simulink model "ISP"  (R2022b)
settings: configuration reference "ERT" (kept outside this file)
undefined symbols (not defined in the file): DFC, ECM, facAdc2ubr_C, facNCtrlRateLim_C, FID, IsRate_C, ki_C, tauIsHeatPnt_C, tauOscDrvTrn_C, tInvMax_C, tInvMin_C, trqDmpSta_C, Ts_10ms, Ts_1ms, tStrMax_C, tStrMin_C, ubrMax_C, ubrMin_C, vdd5Max_C, vdd5Min_C
libraries: simulink x18, DSMLib x17, MathLib x10
settings Model: Creator=M00039784  LastModifiedBy=M00039784
settings ConfigSetRef: SourceName=ERT  SourceLocation=Base Workspace

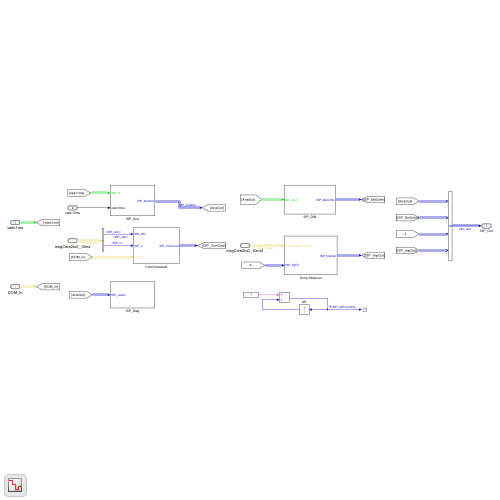
[thumbnail: Simulink's stored preview of the top-level diagram]
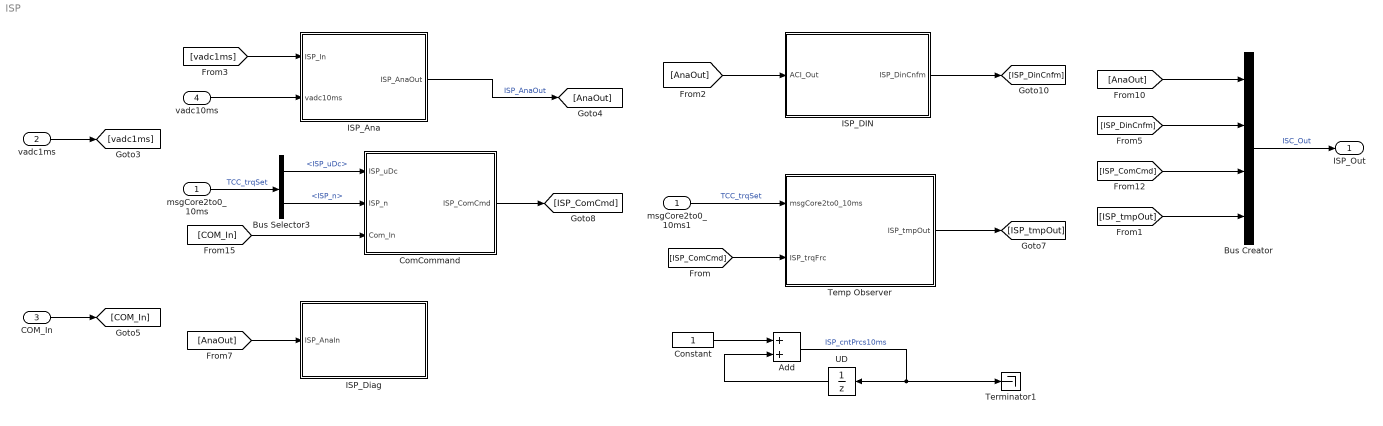
== system ISP ==
  msgCore2to0_10ms : Inport  OutDataTypeStr=Bus: Sig10ms20ST
  vadc1ms : Inport  Port=2  OutDataTypeStr=Bus: Core0_ADC_1ms
  COM_In : Inport  Port=3  OutDataTypeStr=Bus: Core0_COM_Out
  vadc10ms : Inport  Port=4  OutDataTypeStr=Bus: Core0_ADC_10ms
  Add : Sum
  Bus Creator : BusCreator  Inputs=4  OutDataTypeStr=Bus: Core0_ISP_Out  NonVirtualBus=on
  Bus Selector3 : BusSelector  OutputSignals=ISP_uDc,ISP_n
  ComCommand : Subsystem
  Constant : Constant  OutDataTypeStr=uint16
  ISP_Ana : Subsystem
  ISP_DIN : Subsystem
  ISP_Diag : Subsystem
  Temp Observer : Subsystem
  Terminator1 : Terminator
  UD : UnitDelay  InitialCondition=false  SampleTime=Ts_10ms  HasFrameUpgradeWarning=on
  msgCore2to0_10ms1 : InportShadow  OutDataTypeStr=Bus: Sig10ms20ST
  ISP_Out : Outport  OutDataTypeStr=Bus: Core0_ISP_Out  VectorParamsAs1DForOutWhenUnconnected=off  BusOutputAsStruct=on
  wires:
  UD/1 -> Add/2
  [ISP_tmpOut] -> Bus Creator/4
  vadc1ms/1 -> [vadc1ms]
  COM_In/1 -> [COM_In]
  [COM_In] -> ComCommand/3(Com_In)
  ISP_DIN/1(ISP_DinCnfm) -> [ISP_DinCnfm]
  ComCommand/1(ISP_ComCmd) -> [ISP_ComCmd]
  [AnaOut] -> ISP_Diag/1(ISP_AnaIn)
  Bus Selector3/1 -> ComCommand/1(ISP_uDc)  "<ISP_uDc>"
  Add/1 -> Terminator1/1, UD/1  "ISP_cntPrcs10ms"
  Bus Creator/1 -> ISP_Out/1  "ISC_Out"
  Constant/1 -> Add/1
  [ISP_ComCmd] -> Temp Observer/2(ISP_trqFrc)
  [vadc1ms] -> ISP_Ana/1(ISP_In)
  Temp Observer/1(ISP_tmpOut) -> [ISP_tmpOut]
  [ISP_DinCnfm] -> Bus Creator/2
  ISP_Ana/1(ISP_AnaOut) -> [AnaOut]  "ISP_AnaOut"
  Bus Selector3/2 -> ComCommand/2(ISP_n)  "<ISP_n>"
  [ISP_ComCmd] -> Bus Creator/3
  [AnaOut] -> ISP_DIN/1(ACI_Out)
  [AnaOut] -> Bus Creator/1
  msgCore2to0_10ms/1 -> Bus Selector3/1  "TCC_trqSet"
  msgCore2to0_10ms1/1 -> Temp Observer/1(msgCore2to0_10ms)  "TCC_trqSet"
  vadc10ms/1 -> ISP_Ana/2(vadc10ms)

== system ISP/ComCommand ==
  ISP_uDc : Inport
  ISP_n : Inport  Port=2
  Com_In : Inport  Port=3
  ActiveDampingParameters : Subsystem
  Bus Creator1 : BusCreator  Inputs=6  OutDataTypeStr=Bus: Core0_ISP_ComCmd
  CmdProcess : Subsystem
  ControlParameters : Subsystem
  Udc ControlParameters : Subsystem
  ISP_ComCmd : Outport  VectorParamsAs1DForOutWhenUnconnected=off
  wires:
  ControlParameters/1(ISP_ctrlParax) -> Bus Creator1/5  "ISP_ctrlParax"
  CmdProcess/3(ISC_setx) -> Bus Creator1/4  "ISP_cmdx"
  CmdProcess/1(ISP_stModeReq) -> Bus Creator1/2  "ISP_stModeReq"
  CmdProcess/2(ISP_trqX) -> Bus Creator1/3  "ISP_trqx"
  Udc ControlParameters/1(ISP_Dcx) -> Bus Creator1/1  "ISP_Dcx"
  Bus Creator1/1 -> ISP_ComCmd/1  "ISP_ComCmd"
  Com_In/1 -> CmdProcess/1(Com_In), ControlParameters/1(COM), ActiveDampingParameters/1(COM), Udc ControlParameters/2(COM)
  ISP_n/1 -> CmdProcess/2(ISp_n)
  ISP_uDc/1 -> Udc ControlParameters/1(uDc)
  ActiveDampingParameters/1(ISP_ActDmpCtrl) -> Bus Creator1/6

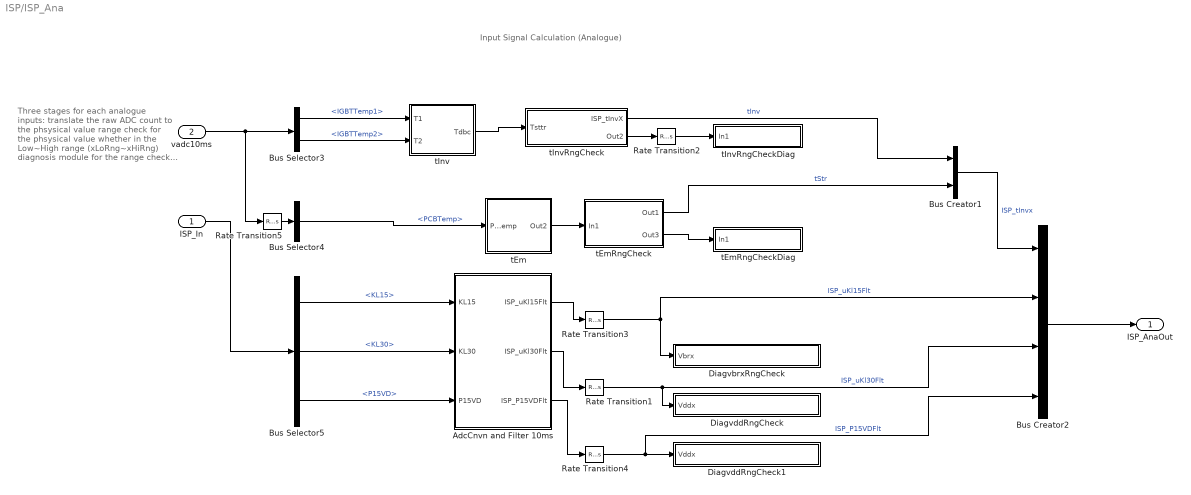
== system ISP/ISP_Ana ==
  note: Input Signal Calculation (Analogue)
  note: Three stages for each analogue inputs:
      | translate the raw ADC count to the phsysical value
      | range check for the phsysical value whether in the Low~High range (xLoRng~xHiRng)
      | diagnosis module for the range check result. The module is in Cyan background
  ISP_In : Inport
  vadc10ms : Inport  Port=2
  AdcCnvn and Filter 10ms : Subsystem  TreatAsAtomicUnit=on  SystemSampleTime=Ts_1ms
  Bus Creator1 : BusCreator  Inputs=2  OutDataTypeStr=Bus: Core0_ISP_tInvx
  Bus Creator2 : BusCreator  Inputs=4  OutDataTypeStr=Bus: Core0_ISP_AnaOut
  Bus Selector3 : BusSelector  OutputSignals=IGBTTemp1,IGBTTemp2
  Bus Selector4 : BusSelector  OutputSignals=PCBTemp
  Bus Selector5 : BusSelector  OutputSignals=KL15,KL30,P15VD
  DiagvbrxRngCheck : Subsystem
  DiagvddRngCheck : Subsystem
  DiagvddRngCheck1 : Subsystem
  Rate Transition1 : RateTransition  InitialCondition=ECM.Init  OutPortSampleTime=Ts_10ms
  Rate Transition2 : RateTransition
  Rate Transition3 : RateTransition  InitialCondition=ECM.Init  OutPortSampleTime=Ts_10ms
  Rate Transition4 : RateTransition  InitialCondition=ECM.Init  OutPortSampleTime=Ts_10ms
  Rate Transition5 : RateTransition
  tEm : Subsystem  TreatAsAtomicUnit=on  SystemSampleTime=Ts_10ms
  tEmRngCheck : Subsystem
  tEmRngCheckDiag : Subsystem  TreatAsAtomicUnit=on  SystemSampleTime=Ts_10ms
  tInv : Subsystem  TreatAsAtomicUnit=on  SystemSampleTime=Ts_10ms
  tInvRngCheck : Subsystem
  tInvRngCheckDiag : Subsystem  TreatAsAtomicUnit=on  SystemSampleTime=Ts_10ms
  ISP_AnaOut : Outport  OutDataTypeStr=Bus: Core0_ISP_AnaOut  VectorParamsAs1DForOutWhenUnconnected=off
  wires:
  tEmRngCheck/2(Out3) -> tEmRngCheckDiag/1(In1)
  Rate Transition2/1 -> tInvRngCheckDiag/1(In1)
  tInvRngCheck/2(Out2) -> Rate Transition2/1
  tInvRngCheck/1(ISP_tInvX) -> Bus Creator1/1  "tInv"
  tInv/1(Tdbc) -> tInvRngCheck/1(Tsttr)
  tEm/1(Out2) -> tEmRngCheck/1(In1)
  ISP_In/1 -> Bus Selector5/1
  Bus Creator1/1 -> Bus Creator2/1  "ISP_tInvx"
  tEmRngCheck/1(Out1) -> Bus Creator1/2  "tStr"
  Bus Selector3/2 -> tInv/2(T2)  "<IGBTTemp2>"
  Bus Selector3/1 -> tInv/1(T1)  "<IGBTTemp1>"
  Bus Selector4/1 -> tEm/1(PCBTemp)  "<PCBTemp>"
  Bus Creator2/1 -> ISP_AnaOut/1
  AdcCnvn and Filter 10ms/1(ISP_uKl15Flt) -> Rate Transition3/1
  Rate Transition3/1 -> DiagvbrxRngCheck/1(Vbrx), Bus Creator2/2  "ISP_uKl15Flt"
  Rate Transition1/1 -> Bus Creator2/3, DiagvddRngCheck/1(Vddx)  "ISP_uKl30Flt"
  Rate Transition5/1 -> Bus Selector4/1
  vadc10ms/1 -> Rate Transition5/1, Bus Selector3/1
  Bus Selector5/1 -> AdcCnvn and Filter 10ms/1(KL15)  "<KL15>"
  Bus Selector5/2 -> AdcCnvn and Filter 10ms/2(KL30)  "<KL30>"
  AdcCnvn and Filter 10ms/2(ISP_uKl30Flt) -> Rate Transition1/1
  Bus Selector5/3 -> AdcCnvn and Filter 10ms/3(P15VD)  "<P15VD>"
  AdcCnvn and Filter 10ms/3(ISP_P15VDFlt) -> Rate Transition4/1
  Rate Transition4/1 -> Bus Creator2/4, DiagvddRngCheck1/1(Vddx)  "ISP_P15VDFlt"

== system ISP/ISP_DIN ==
  ACI_Out : Inport
  DigSigCnfm : Subsystem
  ISP_DinCnfm : Outport  VectorParamsAs1DForOutWhenUnconnected=off
  wires:
  DigSigCnfm/1(Outport) -> ISP_DinCnfm/1  "ISP_DinCnfm"
  ACI_Out/1 -> DigSigCnfm/1(ISP_Din)

== system ISP/ISP_Diag ==
  ISP_AnaIn : Inport

== system ISP/Temp Observer ==
  msgCore2to0_10ms : Inport
  ISP_trqFrc : Inport  Port=2
  Bus Creator : BusCreator  Inputs=4
  Display1 : Display
  IGBT Tstr/Trtr Observer : Subsystem
  ISC_tmpMaxCap : Constant  Value=105  OutDataTypeStr=single
  ISC_tmpMaxRtr : Constant  Value=120  OutDataTypeStr=single
  IsHeatPoint : Subsystem
  ISP_tmpOut : Outport  OutDataTypeStr=Bus: Core0_ISP_tmpOut  VectorParamsAs1DForOutWhenUnconnected=off
  wires:
  msgCore2to0_10ms/1 -> IsHeatPoint/1(msgCore2to0_10ms), IGBT Tstr/Trtr Observer/1(msgCore2to0_10ms)
  ISP_trqFrc/1 -> IGBT Tstr/Trtr Observer/2(trqFrc)
  IGBT Tstr/Trtr Observer/2(ISP_LossMotor) -> Display1/1  "ISP_LossMotor"
  Bus Creator/1 -> ISP_tmpOut/1  "ISP_tmpOut"
  ISC_tmpMaxRtr/1 -> Bus Creator/2  "ISP_tmpMaxRtr"
  ISC_tmpMaxCap/1 -> Bus Creator/3  "ISP_tmpMaxCap"
  IGBT Tstr/Trtr Observer/1(ISP_tmpMaxStr) -> Bus Creator/1  "ISP_tmpMaxStr"
  IsHeatPoint/1(ISP_ratIsHeatPnt) -> Bus Creator/4

== system ISP/ComCommand/ActiveDampingParameters ==
  COM : Inport
  Bus Selector18 : BusSelector  OutputSignals=Com_MSG06
  ISP_ActDmpCtrl : Outport  OutDataTypeStr=Bus: Com_MSG06  VectorParamsAs1DForOutWhenUnconnected=off
  wires:
  Bus Selector18/1 -> ISP_ActDmpCtrl/1  "<Com_MSG06>"
  COM/1 -> Bus Selector18/1

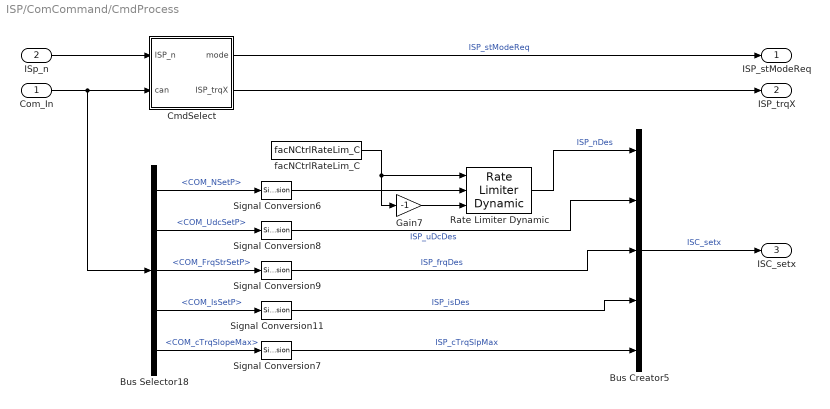
== system ISP/ComCommand/CmdProcess ==
  Com_In : Inport
  ISp_n : Inport  Port=2
  Bus Creator5 : BusCreator  Inputs=5  OutDataTypeStr=Bus: Core0_ISP_cmdx
  Bus Selector18 : BusSelector  OutputSignals=Com_MSG04.COM_NSetP,Com_MSG04.COM_UdcSetP,Com_MSG05.COM_FrqStrSetP,Com_MSG05.COM_IsSetP,Com_MSG03.COM_cTrqSlopeMax
  CmdSelect : Subsystem
      settings: AttributesFormatString=|
      | -------------------------------
      | Select the command source.
      | Sim signals default.
  Gain7 : Gain  Gain=-1  ParamDataTypeStr=single
  Rate Limiter Dynamic : simulink/Discontinuities/Rate Limiter Dynamic
  Signal Conversion{6..9,11} (5 alike) : SignalConversion  OverrideOpt=off
  facNCtrlRateLim_C : Constant  Value=facNCtrlRateLim_C  OutDataTypeStr=single  SampleTime=-1
  ISP_stModeReq : Outport  VectorParamsAs1DForOutWhenUnconnected=off
  ISP_trqX : Outport  Port=2  VectorParamsAs1DForOutWhenUnconnected=off
  ISC_setx : Outport  Port=3  OutDataTypeStr=Bus: Core0_ISP_cmdx  VectorParamsAs1DForOutWhenUnconnected=off
  wires:
  Com_In/1 -> Bus Selector18/1, CmdSelect/2(can)
  CmdSelect/1(mode) -> ISP_stModeReq/1  "ISP_stModeReq"
  CmdSelect/2(ISP_trqX) -> ISP_trqX/1
  Bus Selector18/1 -> Signal Conversion6/1  "<COM_NSetP>"
  Bus Selector18/3 -> Signal Conversion9/1  "<COM_FrqStrSetP>"
  Bus Selector18/2 -> Signal Conversion8/1  "<COM_UdcSetP>"
  Signal Conversion8/1 -> Bus Creator5/2  "ISP_uDcDes"
  Signal Conversion9/1 -> Bus Creator5/3  "ISP_frqDes"
  Rate Limiter Dynamic/1 -> Bus Creator5/1  "ISP_nDes"
  Bus Creator5/1 -> ISC_setx/1  "ISC_setx"
  Bus Selector18/4 -> Signal Conversion11/1  "<COM_IsSetP>"
  Signal Conversion11/1 -> Bus Creator5/4  "ISP_isDes"
  Bus Selector18/5 -> Signal Conversion7/1  "<COM_cTrqSlopeMax>"
  Signal Conversion7/1 -> Bus Creator5/5  "ISP_cTrqSlpMax"
  ISp_n/1 -> CmdSelect/1(ISP_n)
  Gain7/1 -> Rate Limiter Dynamic/3
  Signal Conversion6/1 -> Rate Limiter Dynamic/2
  facNCtrlRateLim_C/1 -> Rate Limiter Dynamic/1, Gain7/1

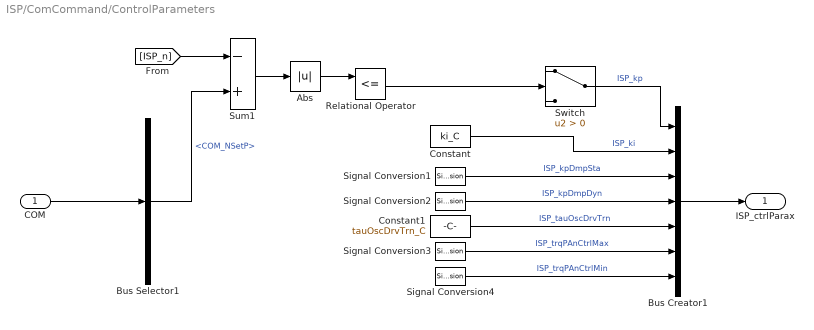
== system ISP/ComCommand/ControlParameters ==
  COM : Inport
  Abs : Abs  SaturateOnIntegerOverflow=off
  Bus Creator1 : BusCreator  Inputs=7  OutDataTypeStr=Bus: Core0_ISP_ctrlParax
  Bus Selector1 : BusSelector  OutputSignals=Com_MSG04.COM_NSetP
  Constant : Constant  Value=ki_C
  Constant1 : Constant  Value=tauOscDrvTrn_C
  Relational Operator : RelationalOperator  Operator=<=  OutDataTypeStr=boolean  RndMeth=Simplest  InputSameDT=off
  Signal Conversion{1..4} (4 alike) : SignalConversion  OverrideOpt=off
  Sum1 : Sum  Inputs=-+  InputSameDT=on  SaturateOnIntegerOverflow=on  OutDataTypeStr=Inherit: Same as first input
  Switch : Switch  Criteria=u2 > Threshold  SaturateOnIntegerOverflow=off  InputSameDT=off
  ISP_ctrlParax : Outport  VectorParamsAs1DForOutWhenUnconnected=off
  wires:
  Bus Creator1/1 -> ISP_ctrlParax/1
  Relational Operator/1 -> Switch/2
  Signal Conversion1/1 -> Bus Creator1/3  "ISP_kpDmpSta"
  Switch/1 -> Bus Creator1/1  "ISP_kp"
  COM/1 -> Bus Selector1/1
  Signal Conversion3/1 -> Bus Creator1/6  "ISP_trqPAnCtrlMax"
  Signal Conversion2/1 -> Bus Creator1/4  "ISP_kpDmpDyn"
  Constant/1 -> Bus Creator1/2  "ISP_ki"
  Signal Conversion4/1 -> Bus Creator1/7  "ISP_trqPAnCtrlMin"
  Abs/1 -> Relational Operator/1
  Bus Selector1/1 -> Sum1/2  "<COM_NSetP>"
  [ISP_n] -> Sum1/1
  Sum1/1 -> Abs/1
  Constant1/1 -> Bus Creator1/5  "ISP_tauOscDrvTrn"

== system ISP/ComCommand/Udc ControlParameters ==
  note: <TODO> dclink power calculation
  uDc : Inport
  COM : Inport  Port=2
  Bus Creator1 : BusCreator  Inputs=6  OutDataTypeStr=Bus: Core0_ISP_Dcx
  Constant : Constant  Value=3000  OutDataTypeStr=single
  Signal Conversion{1..4} (4 alike) : SignalConversion  OverrideOpt=off
  ISP_Dcx : Outport  OutDataTypeStr=Bus: Core0_ISP_Dcx  VectorParamsAs1DForOutWhenUnconnected=off
  wires:
  Signal Conversion4/1 -> Bus Creator1/6  "uDcMin"
  Signal Conversion2/1 -> Bus Creator1/4  "iDcMin"
  Signal Conversion3/1 -> Bus Creator1/5  "uDcMax"
  COM/1 -> ?
  Signal Conversion1/1 -> Bus Creator1/3  "iDcMax"
  Bus Creator1/1 -> ISP_Dcx/1
  uDc/1 -> Bus Creator1/2
  Constant/1 -> Bus Creator1/1  "pwrDc"

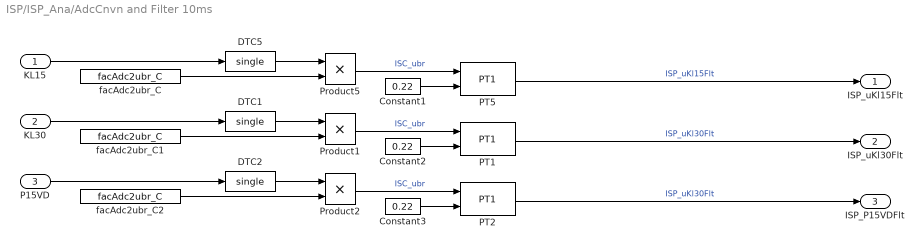
== system ISP/ISP_Ana/AdcCnvn and Filter 10ms ==
  KL15 : Inport
  KL30 : Inport  Port=2
  P15VD : Inport  Port=3
  Constant1 : Constant  Value=0.22  OutDataTypeStr=single
  Constant2 : Constant  Value=0.22  OutDataTypeStr=single
  Constant3 : Constant  Value=0.22  OutDataTypeStr=single
  DTC1 : DataTypeConversion  OutDataTypeStr=single  SaturateOnIntegerOverflow=off  RndMeth=Floor
  DTC2 : DataTypeConversion  OutDataTypeStr=single  SaturateOnIntegerOverflow=off  RndMeth=Floor
  DTC5 : DataTypeConversion  OutDataTypeStr=single  SaturateOnIntegerOverflow=off  RndMeth=Floor
  PT1 : MathLib/PT1  SystemSampleTime=-1  VariantActivationTime=update diagram  Latency=0  AutoFrameSizeCalculation=off
  PT2 : MathLib/PT1  SystemSampleTime=-1  VariantActivationTime=update diagram  Latency=0  AutoFrameSizeCalculation=off
  PT5 : MathLib/PT1  SystemSampleTime=-1  VariantActivationTime=update diagram  Latency=0  AutoFrameSizeCalculation=off
  Product1 : Product  OutDataTypeStr=single
  Product2 : Product  OutDataTypeStr=single
  Product5 : Product  OutDataTypeStr=single
  facAdc2ubr_C : Constant  Value=facAdc2ubr_C
      mask Display:
      | tmpx = get_param(gcbh,'Value');
      | a= evalin('base',[tmpx,'.Value;']);
      | disp([tmpx,': ',num2str(a)]);
  facAdc2ubr_C1 : Constant  Value=facAdc2ubr_C
      mask Display:
      | tmpx = get_param(gcbh,'Value');
      | a= evalin('base',[tmpx,'.Value;']);
      | disp([tmpx,': ',num2str(a)]);
  facAdc2ubr_C2 : Constant  Value=facAdc2ubr_C
      mask Display:
      | tmpx = get_param(gcbh,'Value');
      | a= evalin('base',[tmpx,'.Value;']);
      | disp([tmpx,': ',num2str(a)]);
  ISP_uKl15Flt : Outport
  ISP_uKl30Flt : Outport  Port=2
  ISP_P15VDFlt : Outport  Port=3
  wires:
  Product5/1 -> PT5/1  "ISC_ubr"
  KL15/1 -> DTC5/1
  facAdc2ubr_C/1 -> Product5/2
  DTC5/1 -> Product5/1
  Constant1/1 -> PT5/2
  PT5/1 -> ISP_uKl15Flt/1  "ISP_uKl15Flt"
  Constant2/1 -> PT1/2
  Product1/1 -> PT1/1  "ISC_ubr"
  DTC1/1 -> Product1/1
  facAdc2ubr_C1/1 -> Product1/2
  KL30/1 -> DTC1/1
  PT1/1 -> ISP_uKl30Flt/1  "ISP_uKl30Flt"
  facAdc2ubr_C2/1 -> Product2/2
  Product2/1 -> PT2/1  "ISC_ubr"
  DTC2/1 -> Product2/1
  Constant3/1 -> PT2/2
  P15VD/1 -> DTC2/1
  PT2/1 -> ISP_P15VDFlt/1  "ISP_uKl30Flt"

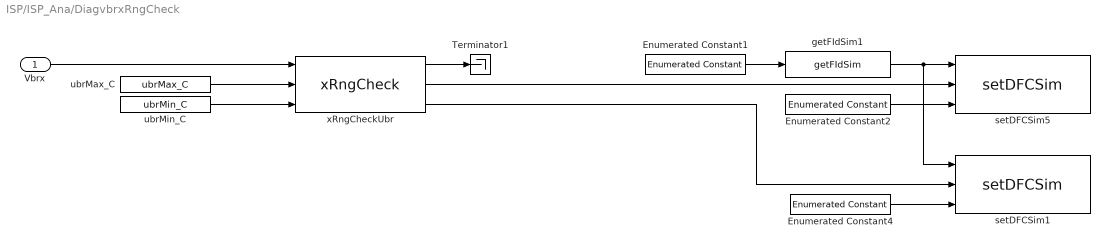
== system ISP/ISP_Ana/DiagvbrxRngCheck ==
  Vbrx : Inport
  Enumerated Constant1 : simulink/Sources/Enumerated Constant  OutDataTypeStr=Enum: FID  Value=FID.DiagUbrHiLoRng  SampleTime=inf
  Enumerated Constant2 : simulink/Sources/Enumerated Constant  OutDataTypeStr=Enum: DFC  Value=DFC.UbrHiRng  SampleTime=inf
  Enumerated Constant4 : simulink/Sources/Enumerated Constant  OutDataTypeStr=Enum: DFC  Value=DFC.UbrLoRng  SampleTime=inf
  Terminator1 : Terminator
  getFIdSim1 : DSMLib/getFIdSim  SystemSampleTime=-1  VariantActivationTime=update diagram  Latency=0  AutoFrameSizeCalculation=off
  setDFCSim1 : DSMLib/setDFCSim  SystemSampleTime=-1  VariantActivationTime=update diagram  Latency=0  AutoFrameSizeCalculation=off
  setDFCSim5 : DSMLib/setDFCSim  SystemSampleTime=-1  VariantActivationTime=update diagram  Latency=0  AutoFrameSizeCalculation=off
  ubrMax_C : Constant  Value=ubrMax_C
      mask Display:
      | tmpx = get_param(gcbh,'Value');
      | a= evalin('base',[tmpx,'.Value;']);
      | disp([tmpx,': ',num2str(a)]);
  ubrMin_C : Constant  Value=ubrMin_C
      mask Display:
      | tmpx = get_param(gcbh,'Value');
      | a= evalin('base',[tmpx,'.Value;']);
      | disp([tmpx,': ',num2str(a)]);
  xRngCheckUbr : MathLib/xRngCheck  SystemSampleTime=-1  VariantActivationTime=update diagram  Latency=0  AutoFrameSizeCalculation=off
  wires:
  ubrMin_C/1 -> xRngCheckUbr/3
  ubrMax_C/1 -> xRngCheckUbr/2
  xRngCheckUbr/2 -> setDFCSim5/2
  Vbrx/1 -> xRngCheckUbr/1
  Enumerated Constant2/1 -> setDFCSim5/3
  Enumerated Constant1/1 -> getFIdSim1/1
  getFIdSim1/1 -> setDFCSim1/1, setDFCSim5/1
  Enumerated Constant4/1 -> setDFCSim1/3
  xRngCheckUbr/3 -> setDFCSim1/2
  xRngCheckUbr/1 -> Terminator1/1

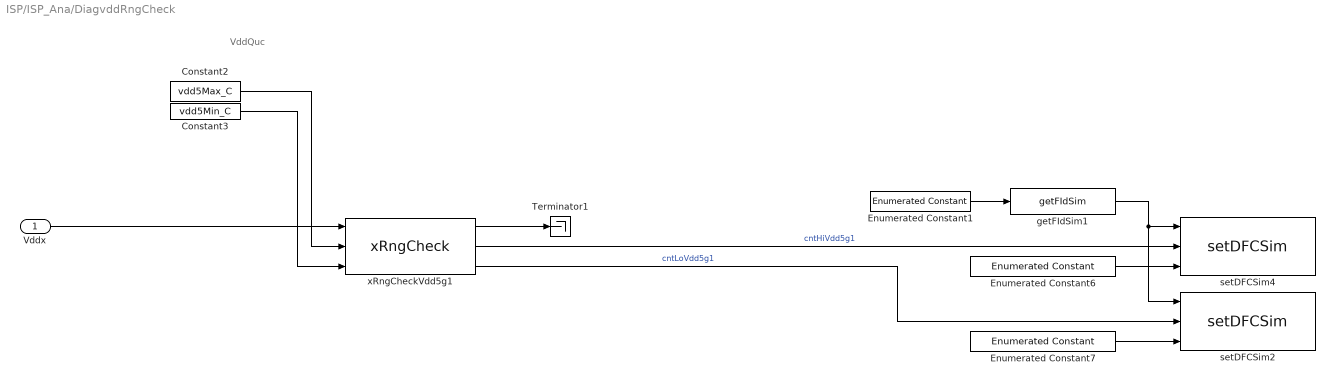
== system ISP/ISP_Ana/DiagvddRngCheck ==
  note: VddQuc
  Vddx : Inport
  Constant2 : Constant  Value=vdd5Max_C
  Constant3 : Constant  Value=vdd5Min_C
  Enumerated Constant1 : simulink/Sources/Enumerated Constant  OutDataTypeStr=Enum: FID  Value=FID.DiagUbrHiLoRng  SampleTime=inf
  Enumerated Constant6 : simulink/Sources/Enumerated Constant  OutDataTypeStr=Enum: DFC  Value=DFC.Vdd5g1HiRng  SampleTime=inf
  Enumerated Constant7 : simulink/Sources/Enumerated Constant  OutDataTypeStr=Enum: DFC  Value=DFC.Vdd5g1LoRng  SampleTime=inf
  Terminator1 : Terminator
  getFIdSim1 : DSMLib/getFIdSim  SystemSampleTime=-1  VariantActivationTime=update diagram  Latency=0  AutoFrameSizeCalculation=off
  setDFCSim2 : DSMLib/setDFCSim  SystemSampleTime=-1  VariantActivationTime=update diagram  Latency=0  AutoFrameSizeCalculation=off
  setDFCSim4 : DSMLib/setDFCSim  SystemSampleTime=-1  VariantActivationTime=update diagram  Latency=0  AutoFrameSizeCalculation=off
  xRngCheckVdd5g1 : MathLib/xRngCheck  SystemSampleTime=-1  VariantActivationTime=update diagram  Latency=0  AutoFrameSizeCalculation=off
  wires:
  Constant2/1 -> xRngCheckVdd5g1/2
  Vddx/1 -> xRngCheckVdd5g1/1
  Constant3/1 -> xRngCheckVdd5g1/3
  xRngCheckVdd5g1/3 -> setDFCSim2/2  "cntLoVdd5g1"
  xRngCheckVdd5g1/2 -> setDFCSim4/2  "cntHiVdd5g1"
  xRngCheckVdd5g1/1 -> Terminator1/1
  Enumerated Constant6/1 -> setDFCSim4/3
  Enumerated Constant7/1 -> setDFCSim2/3
  getFIdSim1/1 -> setDFCSim4/1, setDFCSim2/1
  Enumerated Constant1/1 -> getFIdSim1/1

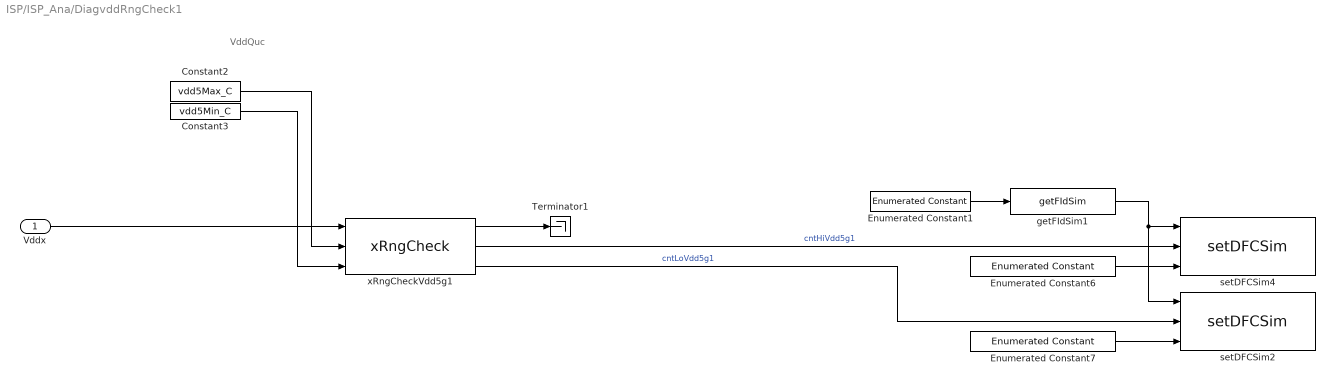
== system ISP/ISP_Ana/DiagvddRngCheck1 ==
  note: VddQuc
  Vddx : Inport
  Constant2 : Constant  Value=vdd5Max_C
  Constant3 : Constant  Value=vdd5Min_C
  Enumerated Constant1 : simulink/Sources/Enumerated Constant  OutDataTypeStr=Enum: FID  Value=FID.DiagUbrHiLoRng  SampleTime=inf
  Enumerated Constant6 : simulink/Sources/Enumerated Constant  OutDataTypeStr=Enum: DFC  Value=DFC.Vdd5g1HiRng  SampleTime=inf
  Enumerated Constant7 : simulink/Sources/Enumerated Constant  OutDataTypeStr=Enum: DFC  Value=DFC.Vdd5g1LoRng  SampleTime=inf
  Terminator1 : Terminator
  getFIdSim1 : DSMLib/getFIdSim  SystemSampleTime=-1  VariantActivationTime=update diagram  Latency=0  AutoFrameSizeCalculation=off
  setDFCSim2 : DSMLib/setDFCSim  SystemSampleTime=-1  VariantActivationTime=update diagram  Latency=0  AutoFrameSizeCalculation=off
  setDFCSim4 : DSMLib/setDFCSim  SystemSampleTime=-1  VariantActivationTime=update diagram  Latency=0  AutoFrameSizeCalculation=off
  xRngCheckVdd5g1 : MathLib/xRngCheck  SystemSampleTime=-1  VariantActivationTime=update diagram  Latency=0  AutoFrameSizeCalculation=off
  wires:
  Constant2/1 -> xRngCheckVdd5g1/2
  Vddx/1 -> xRngCheckVdd5g1/1
  Constant3/1 -> xRngCheckVdd5g1/3
  xRngCheckVdd5g1/3 -> setDFCSim2/2  "cntLoVdd5g1"
  xRngCheckVdd5g1/2 -> setDFCSim4/2  "cntHiVdd5g1"
  xRngCheckVdd5g1/1 -> Terminator1/1
  Enumerated Constant6/1 -> setDFCSim4/3
  Enumerated Constant7/1 -> setDFCSim2/3
  getFIdSim1/1 -> setDFCSim4/1, setDFCSim2/1
  Enumerated Constant1/1 -> getFIdSim1/1

== system ISP/ISP_Ana/tEm ==
  PCBTemp : Inport
  Data Type Conversion : DataTypeConversion  OutDataTypeStr=single  SaturateOnIntegerOverflow=off  RndMeth=Floor
  H : Lookup_n-D  NumberOfTableDimensions=1  DataSpecification=Lookup table object  LookupTableObject=tEmH_T  BreakpointsForDimension1="[1024    2048.0\t3072.0\t4096.0\t5120.0\t6144.0\t7168.0\t8192.0\t9216.0\t10240.0\t11264.0\t12288.0\t13312.0\t14336.0\t15360.0\t16384.0\t17408.0\t18432.0\t19456.0\t20480.0\t21504.0\t22528.0\t23552.0\t24576.0\t25600.0\t26624.0\t27648.0\t28672.0\t29696.0\t30720.0\t31744.0\t32768.0\t33792.0\t34816.0\t35840.0\t36864.0\t37888.0\t38912.0\t39936.0\t40960.0\t41984.0\t43008.0\t44032.0\t45056.0\t46080.0\t47104.0\t48128.0\t49152.0\t50176.0\t51200.0\t52224.0\t53248.0\t54272.0\t55296.0\t56320.0\t57344.0\t58368.0\t59392.0\t60416.0\t61440.0\t62464.0\t63488.0\t64512.0\t65534.0]"  BeginIndexSearchUsingPreviousIndexResult=on  Table="[299.0\t299.0\t270.0\t251.0\t236.0\t225.0\t215.0\t207.0\t200.0\t194.0\t188.0\t183.0\t179.0\t174.0\t170.0\t166.0\t163.0\t159.0\t156.0\t153.0\t150.0\t147.0\t144.0\t141.0\t139.0\t136.0\t134.0\t131.0\t129.0\t126.0\t124.0\t122.0\t120.0\t117.0\t115.0\t113.0\t111.0\t108.0\t106.0\t104.0\t102.0\t99.0\t97.0\t95.0\t92.0\t90.0\t87.0\t85.0\t82.0\t79.0\t77.0\t74.0\t71.0\t67.0\t64.0\t60.0\t56.0\t52.0\t46.0\t40.0\t33.0\t23.0\t8.0\t-59.0]"  ExtrapMethod=Clip  UseLastTableValue=on  InternalRulePriority=Speed  OutDataTypeStr=Inherit: Inherit from 'Table data'  RndMeth=Simplest
  Out2 : Outport  VectorParamsAs1DForOutWhenUnconnected=off
  wires:
  Data Type Conversion/1 -> H/1
  H/1 -> Out2/1
  PCBTemp/1 -> Data Type Conversion/1

== system ISP/ISP_Ana/tEmRngCheck ==
  In1 : Inport
  Bus Creator3 : BusCreator  Inputs=2
  Demux1 : Demux  Outputs=1
  IdcMaxMdl_C : Constant  Value=tStrMax_C
      mask Display:
      | tmpx = get_param(gcbh,'Value');
      | a= evalin('base',[tmpx,'.Value;']);
      | disp([tmpx,': ',num2str(a)]);
  IdcMaxMdl_C1 : Constant  Value=tStrMin_C
      mask Display:
      | tmpx = get_param(gcbh,'Value');
      | a= evalin('base',[tmpx,'.Value;']);
      | disp([tmpx,': ',num2str(a)]);
  xRngCheckU : MathLib/xRngCheck  SystemSampleTime=-1  VariantActivationTime=update diagram  Latency=0  AutoFrameSizeCalculation=off
  Out1 : Outport  VectorParamsAs1DForOutWhenUnconnected=off
  Out3 : Outport  Port=2  VectorParamsAs1DForOutWhenUnconnected=off
  wires:
  Bus Creator3/1 -> Out3/1
  xRngCheckU/3 -> Bus Creator3/2  "cntLoTstr"
  IdcMaxMdl_C/1 -> xRngCheckU/2
  xRngCheckU/2 -> Bus Creator3/1  "cntHiTstr"
  xRngCheckU/1 -> Out1/1
  In1/1 -> Demux1/1
  IdcMaxMdl_C1/1 -> xRngCheckU/3
  Demux1/1 -> xRngCheckU/1

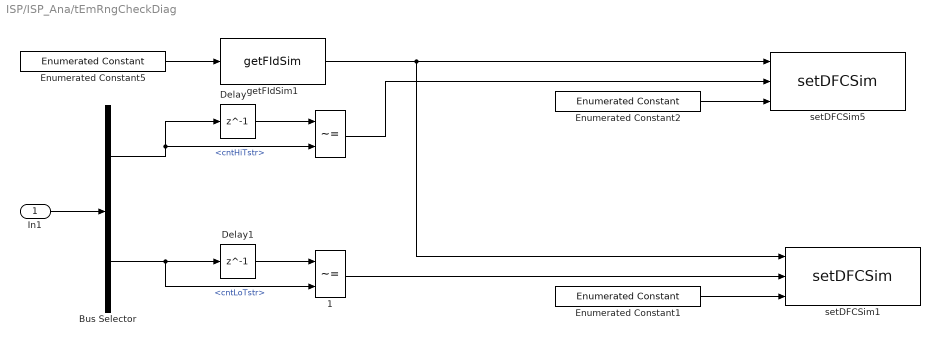
== system ISP/ISP_Ana/tEmRngCheckDiag ==
  In1 : Inport
  " " : RelationalOperator  Operator=~=  OutDataTypeStr=boolean  RndMeth=Simplest  InputSameDT=off
  " 1" : RelationalOperator  Operator=~=  OutDataTypeStr=boolean  RndMeth=Simplest  InputSameDT=off
  Bus Selector : BusSelector  OutputSignals=cntHiTstr,cntLoTstr
  Delay : Delay  DelayLength=1  InitialCondition=0
  Delay1 : Delay  DelayLength=1  InitialCondition=0
  Enumerated Constant1 : simulink/Sources/Enumerated Constant  OutDataTypeStr=Enum: DFC  Value=DFC.tStrLoRng  SampleTime=inf
  Enumerated Constant2 : simulink/Sources/Enumerated Constant  OutDataTypeStr=Enum: DFC  Value=DFC.tStrHiRng  SampleTime=inf
  Enumerated Constant5 : simulink/Sources/Enumerated Constant  OutDataTypeStr=Enum: FID  Value=FID.DiagTstrHiLoRng  SampleTime=inf
  getFIdSim1 : DSMLib/getFIdSim  SystemSampleTime=-1  VariantActivationTime=update diagram  Latency=0  AutoFrameSizeCalculation=off
  setDFCSim1 : DSMLib/setDFCSim  SystemSampleTime=-1  VariantActivationTime=update diagram  Latency=0  AutoFrameSizeCalculation=off
  setDFCSim5 : DSMLib/setDFCSim  SystemSampleTime=-1  VariantActivationTime=update diagram  Latency=0  AutoFrameSizeCalculation=off
  wires:
  Enumerated Constant5/1 -> getFIdSim1/1
  " "/1 -> setDFCSim5/2
  Enumerated Constant2/1 -> setDFCSim5/3
  In1/1 -> Bus Selector/1
  Bus Selector/1 -> Delay/1, " "/2  "<cntHiTstr>"
  Delay/1 -> " "/1
  Enumerated Constant1/1 -> setDFCSim1/3
  getFIdSim1/1 -> setDFCSim5/1, setDFCSim1/1
  Bus Selector/2 -> " 1"/2, Delay1/1  "<cntLoTstr>"
  Delay1/1 -> " 1"/1
  " 1"/1 -> setDFCSim1/2

== system ISP/ISP_Ana/tInv ==
  T1 : Inport
  T2 : Inport  Port=2
  1-D Lookup Table : Lookup_n-D  NumberOfTableDimensions=1  DataSpecification=Lookup table object  LookupTableObject=tInvNtc_T  BreakpointsForDimension1="[688.0\t752.0\t816.0\t880.0\t960.0\t1056.0\t1152.0\t1264.0\t1392.0\t1520.0\t1680.0\t1856.0\t2048.0\t2272.0\t2512.0\t2800.0\t3120.0\t3488.0\t3904.0\t4368.0\t4896.0\t5504.0\t6208.0\t6992.0\t7888.0\t8912.0\t10064.0\t11376.0\t12848.0\t14512.0\t16352.0\t18384.0\t20608.0\t23008.0\t25600.0\t28304.0\t31136.0\t34000.0\t36880.0\t39696.0\t42384.0\t44928.0\t47264.0\t49360.0\t51200.0\t52800.0\t54160.0\t55280.0\t56208.0\t56944.0\t57536.0]"  BeginIndexSearchUsingPreviousIndexResult=on  Table="[200.0\t195.0\t190.0\t185.0\t180.0\t175.0\t170.0\t165.0\t160.0\t155.0\t150.0\t145.0\t140.0\t135.0\t130.0\t125.0\t120.0\t115.0\t110.0\t105.0\t100.0\t95.0\t90.0\t85.0\t80.0\t75.0\t70.0\t65.0\t60.0\t55.0\t50.0\t45.0\t40.0\t35.0\t30.0\t25.0\t20.0\t15.0\t10.0\t5.0\t0.0\t-5.0\t-10.0\t-15.0\t-20.0\t-25.0\t-30.0\t-35.0\t-40.0\t-45.0\t-50.0]"  ExtrapMethod=Clip  UseLastTableValue=on  InternalRulePriority=Speed  OutDataTypeStr=Inherit: Inherit from 'Table data'  RndMeth=Simplest
  Data Type Conversion : DataTypeConversion  OutDataTypeStr=single  SaturateOnIntegerOverflow=off  RndMeth=Floor
  Saturation : Saturate  UpperLimit=255  LowerLimit=0
  Vector Concatenate : Concatenate
  Tdbc : Outport  VectorParamsAs1DForOutWhenUnconnected=off
  wires:
  1-D Lookup Table/1 -> Tdbc/1
  Data Type Conversion/1 -> Saturation/1
  Vector Concatenate/1 -> Data Type Conversion/1
  T1/1 -> Vector Concatenate/1
  T2/1 -> Vector Concatenate/2
  Saturation/1 -> 1-D Lookup Table/1

== system ISP/ISP_Ana/tInvRngCheck ==
  Tsttr : Inport
  Bus Creator1 : BusCreator  Inputs=2  OutDataTypeStr=Bus: Core0_tInv
  Bus Creator2 : BusCreator  Inputs=4
  Constant2 : Constant  Value=tInvMax_C
  Constant3 : Constant  Value=tInvMin_C
  Demux1 : Demux  Outputs=2
  xRngCheckU : MathLib/xRngCheck  SystemSampleTime=-1  VariantActivationTime=update diagram  Latency=0  AutoFrameSizeCalculation=off
  xRngCheckV : MathLib/xRngCheck  SystemSampleTime=-1  VariantActivationTime=update diagram  Latency=0  AutoFrameSizeCalculation=off
  ISP_tInvX : Outport  VectorParamsAs1DForOutWhenUnconnected=off
  Out2 : Outport  Port=2  VectorParamsAs1DForOutWhenUnconnected=off
  wires:
  Bus Creator2/1 -> Out2/1
  Constant3/1 -> xRngCheckV/3, xRngCheckU/3
  Tsttr/1 -> Demux1/1
  xRngCheckV/3 -> Bus Creator2/4  "cntLoTinvV"
  xRngCheckV/2 -> Bus Creator2/3  "cntHiTinvV"
  Bus Creator1/1 -> ISP_tInvX/1
  xRngCheckV/1 -> Bus Creator1/2  "ISP_tDbcInvV"
  xRngCheckU/2 -> Bus Creator2/1  "cntHiTinvU"
  xRngCheckU/3 -> Bus Creator2/2  "cntLoTinvU"
  xRngCheckU/1 -> Bus Creator1/1  "ISP_tDbcInvU"
  Constant2/1 -> xRngCheckV/2, xRngCheckU/2
  Demux1/2 -> xRngCheckV/1
  Demux1/1 -> xRngCheckU/1

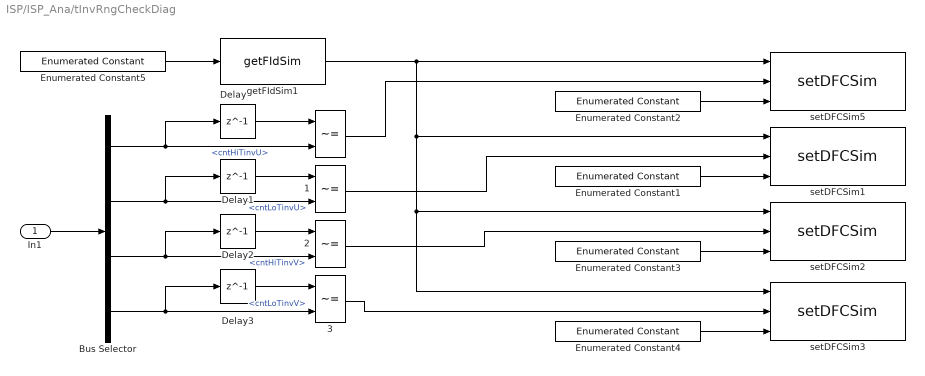
== system ISP/ISP_Ana/tInvRngCheckDiag ==
  In1 : Inport
   {,1..3} (4 alike) : RelationalOperator  Operator=~=  OutDataTypeStr=boolean  RndMeth=Simplest  InputSameDT=off
  Bus Selector : BusSelector  OutputSignals=cntHiTinvU,cntLoTinvU,cntHiTinvV,cntLoTinvV
  Delay{,1..3} (4 alike) : Delay  DelayLength=1  InitialCondition=0
  Enumerated Constant1 : simulink/Sources/Enumerated Constant  OutDataTypeStr=Enum: DFC  Value=DFC.tInvULoRng  SampleTime=inf
  Enumerated Constant2 : simulink/Sources/Enumerated Constant  OutDataTypeStr=Enum: DFC  Value=DFC.tInvUHiRng  SampleTime=inf
  Enumerated Constant3 : simulink/Sources/Enumerated Constant  OutDataTypeStr=Enum: DFC  Value=DFC.tInvVHiRng  SampleTime=inf
  Enumerated Constant4 : simulink/Sources/Enumerated Constant  OutDataTypeStr=Enum: DFC  Value=DFC.tInvVLoRng  SampleTime=inf
  Enumerated Constant5 : simulink/Sources/Enumerated Constant  OutDataTypeStr=Enum: FID  Value=FID.DiagTinvHiLoRng  SampleTime=inf
  getFIdSim1 : DSMLib/getFIdSim  SystemSampleTime=-1  VariantActivationTime=update diagram  Latency=0  AutoFrameSizeCalculation=off
  setDFCSim{1..3,5} (4 alike) : DSMLib/setDFCSim  SystemSampleTime=-1  VariantActivationTime=update diagram  Latency=0  AutoFrameSizeCalculation=off
  wires:
  " 3"/1 -> setDFCSim3/2
  " 2"/1 -> setDFCSim2/2
  " 1"/1 -> setDFCSim1/2
  Delay3/1 -> " 3"/1
  Bus Selector/4 -> Delay3/1, " 3"/2  "<cntLoTinvV>"
  Delay2/1 -> " 2"/1
  Bus Selector/3 -> Delay2/1, " 2"/2  "<cntHiTinvV>"
  Delay1/1 -> " 1"/1
  Bus Selector/2 -> Delay1/1, " 1"/2  "<cntLoTinvU>"
  getFIdSim1/1 -> setDFCSim5/1, setDFCSim1/1, setDFCSim2/1, setDFCSim3/1
  Enumerated Constant4/1 -> setDFCSim3/3
  Enumerated Constant3/1 -> setDFCSim2/3
  Enumerated Constant1/1 -> setDFCSim1/3
  Delay/1 -> " "/1
  Bus Selector/1 -> " "/2, Delay/1  "<cntHiTinvU>"
  In1/1 -> Bus Selector/1
  Enumerated Constant2/1 -> setDFCSim5/3
  " "/1 -> setDFCSim5/2
  Enumerated Constant5/1 -> getFIdSim1/1

== system ISP/ISP_DIN/DigSigCnfm ==
  ISP_Din : Inport
  Constant : Constant  Value=4.5
  Equal : RelationalOperator  OutDataTypeStr=boolean  RndMeth=Simplest  InputSameDT=off
  KL15 Confirm : MATLAB Function
  Rate Transition : RateTransition  OutPortSampleTime=Ts_10ms
  Sel : BusSelector  OutputSignals=ISP_uKl15Flt
  Outport : Outport
  wires:
  ISP_Din/1 -> Sel/1
  Sel/1 -> Equal/1  "<ISP_uKl15Flt>"
  KL15 Confirm/1(KL15Cnfm) -> Rate Transition/1  "ISP_bKl15Cnfm"
  Rate Transition/1 -> Outport/1
  Equal/1 -> KL15 Confirm/1(KL15_In)
  Constant/1 -> Equal/2

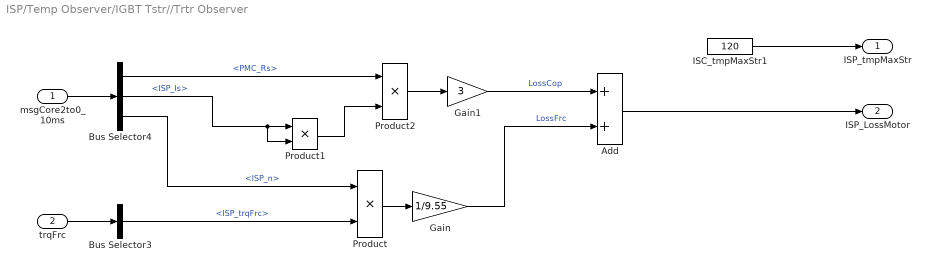
== system ISP/Temp Observer/IGBT Tstr//Trtr Observer ==
  msgCore2to0_10ms : Inport
  trqFrc : Inport  Port=2
  Add : Sum
  Bus Selector3 : BusSelector  OutputSignals=ISP_trqx.ISP_trqFrc
  Bus Selector4 : BusSelector  OutputSignals=PMC_Rs,ISP_Is,ISP_n
  Gain : Gain  Gain=1/9.55
  Gain1 : Gain  Gain=3
  ISC_tmpMaxStr1 : Constant  Value=120  OutDataTypeStr=single
  Product : Product
  Product1 : Product
  Product2 : Product
  ISP_tmpMaxStr : Outport  VectorParamsAs1DForOutWhenUnconnected=off
  ISP_LossMotor : Outport  Port=2  VectorParamsAs1DForOutWhenUnconnected=off
  wires:
  msgCore2to0_10ms/1 -> Bus Selector4/1
  ISC_tmpMaxStr1/1 -> ISP_tmpMaxStr/1
  trqFrc/1 -> Bus Selector3/1
  Product/1 -> Gain/1
  Bus Selector4/2 -> Product1/2, Product1/1  "<ISP_Is>"
  Bus Selector4/1 -> Product2/1  "<PMC_Rs>"
  Product1/1 -> Product2/2
  Product2/1 -> Gain1/1
  Gain1/1 -> Add/1  "LossCop"
  Gain/1 -> Add/2  "LossFrc"
  Add/1 -> ISP_LossMotor/1
  Bus Selector4/3 -> Product/1  "<ISP_n>"
  Bus Selector3/1 -> Product/2  "<ISP_trqFrc>"

== system ISP/Temp Observer/IsHeatPoint ==
  note: tauIsHearPnt_C = 1000;
      | IsRate_C = 200;
      |
      | 450A can stand 240s
      | 300A can stand 600s
  msgCore2to0_10ms : Inport
  Bus Selector4 : BusSelector  OutputSignals=ISP_Is
  Constant : Constant  Value=single(0.01)/tauIsHeatPnt_C  OutDataTypeStr=single
  Constant1 : Constant  Value=IsRate_C
  Constant2 : Constant  Value=IsRate_C
  Divide : Product  Inputs=*/
  Divide1 : Product  Inputs=*/
  PT1_1 : MathLib/PT1  SystemSampleTime=-1  VariantActivationTime=update diagram  Latency=0  AutoFrameSizeCalculation=off
  Product1 : Product
  Rii : Gain  Gain=100/IsRate_C/IsRate_C
  ISP_ratIsHeatPnt : Outport  VectorParamsAs1DForOutWhenUnconnected=off
  wires:
  Bus Selector4/1 -> Product1/1, Product1/2  "<ISP_Is>"
  msgCore2to0_10ms/1 -> Bus Selector4/1
  Product1/1 -> PT1_1/1
  Constant/1 -> PT1_1/2
  PT1_1/1 -> Divide/1
  Divide1/1 -> ISP_ratIsHeatPnt/1  "ISP_ratIsHeatPnt"
  Constant1/1 -> Divide/2
  Divide/1 -> Divide1/1
  Constant2/1 -> Divide1/2

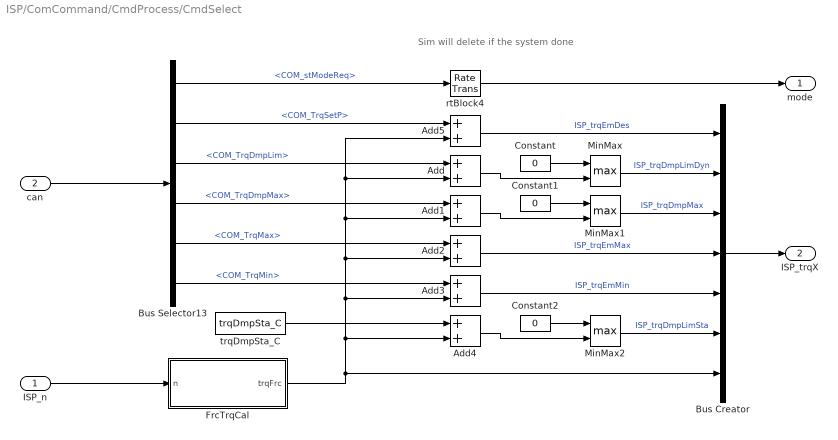
== system ISP/ComCommand/CmdProcess/CmdSelect ==
  note: Sim will delete if the system done
  ISP_n : Inport
  can : Inport  Port=2
  Add{,1..5} (6 alike) : Sum
  Bus Creator : BusCreator  Inputs=7  OutDataTypeStr=Bus: Core0_ISP_trqx
  Bus Selector13 : BusSelector  OutputSignals=Com_MSG04.COM_stModeReq,Com_MSG04.COM_TrqSetP,Com_MSG06.COM_TrqDmpLim,Com_MSG06.COM_TrqDmpMax,Com_MSG03.COM_TrqMax,Com_MSG03.COM_TrqMin
  Constant : Constant  Value=0  OutDataTypeStr=single
  Constant1 : Constant  Value=0  OutDataTypeStr=single
  Constant2 : Constant  Value=0  OutDataTypeStr=single
  FrcTrqCal : Subsystem
  MinMax : MinMax  Function=max  Inputs=2
  MinMax1 : MinMax  Function=max  Inputs=2
  MinMax2 : MinMax  Function=max  Inputs=2
  rtBlock4 : RateTransition  InitialCondition=ECM.Init  OutPortSampleTime=Ts_10ms
  trqDmpSta_C : Constant  Value=trqDmpSta_C  OutDataTypeStr=single
  mode : Outport  VectorParamsAs1DForOutWhenUnconnected=off
  ISP_trqX : Outport  Port=2  OutDataTypeStr=Bus: Core0_ISP_trqx  VectorParamsAs1DForOutWhenUnconnected=off
  wires:
  can/1 -> Bus Selector13/1
  Bus Selector13/1 -> rtBlock4/1  "<COM_stModeReq>"
  Bus Selector13/2 -> Add5/1  "<COM_TrqSetP>"
  Bus Selector13/3 -> Add/1  "<COM_TrqDmpLim>"
  Bus Selector13/4 -> Add1/1  "<COM_TrqDmpMax>"
  Bus Selector13/5 -> Add2/1  "<COM_TrqMax>"
  Bus Selector13/6 -> Add3/1  "<COM_TrqMin>"
  Add5/1 -> Bus Creator/1  "ISP_trqEmDes"
  Add/1 -> MinMax/2
  Add1/1 -> MinMax1/2
  Add3/1 -> Bus Creator/5  "ISP_trqEmMin"
  Bus Creator/1 -> ISP_trqX/1
  MinMax/1 -> Bus Creator/2  "ISP_trqDmpLimDyn"
  MinMax1/1 -> Bus Creator/3  "ISP_trqDmpMax"
  Add2/1 -> Bus Creator/4  "ISP_trqEmMax"
  MinMax2/1 -> Bus Creator/6  "ISP_trqDmpLimSta"
  trqDmpSta_C/1 -> Add4/1
  Constant/1 -> MinMax/1
  Constant1/1 -> MinMax1/1
  Constant2/1 -> MinMax2/1
  Add4/1 -> MinMax2/2
  rtBlock4/1 -> mode/1
  FrcTrqCal/1(trqFrc) -> Add4/2, Add2/2, Add5/2, Add/2, Add1/2, Add3/2, Bus Creator/7
  ISP_n/1 -> FrcTrqCal/1(n)

== system ISP/ComCommand/CmdProcess/CmdSelect/FrcTrqCal ==
  n : Inport
  Abs : Abs  SaturateOnIntegerOverflow=off
  Constant : Constant  Value=0  OutDataTypeStr=single
  FrictionTorque : Lookup_n-D  NumberOfTableDimensions=1  DataSpecification=Lookup table object  LookupTableObject=trqFrcN_T  BreakpointsForDimension1="[0.0\t500.0\t1000.0\t2000.0\t3000.0\t4000.0\t5000.0\t6000.0\t7000.0\t7500.0]"  BeginIndexSearchUsingPreviousIndexResult=on  Table="[2.0\t2.0\t2.25\t2.75\t3.25\t3.75\t4.25\t4.75\t5.25\t5.5]"  ExtrapMethod=Clip  UseLastTableValue=on  InternalRulePriority=Speed  OutDataTypeStr=Inherit: Inherit from 'Table data'  RndMeth=Simplest  InputSameDT=off
  Product : Product  Inputs=3
  Sign : Signum
  trqFrc : Outport  VectorParamsAs1DForOutWhenUnconnected=off
  wires:
  Product/1 -> trqFrc/1  "ISP_trqFrc"
  n/1 -> Sign/1, Abs/1
  Abs/1 -> FrictionTorque/1
  FrictionTorque/1 -> Product/1
  Sign/1 -> Product/2
  Constant/1 -> Product/3

== matlab function ISP/ISP_DIN/DigSigCnfm/KL15 Confirm ==
  data: KL15_In input; KL15Cnfm output
function KL15Cnfm  = fcn(KL15_In)
%
persistent KL15_Last;
persistent KL15_confirm_Last;
if isempty(KL15_Last)
    KL15_Last = true;
    KL15_confirm_Last = true;
end

if (KL15_In==KL15_Last)
    if (KL15_In==true)
        KL15Cnfm = true;
    else
        KL15Cnfm = false;
    end
else
    KL15Cnfm = KL15_confirm_Last;
end

KL15_Last = KL15_In;
KL15_confirm_Last = KL15Cnfm;
